simulink model "TDS_StateSpace"  (R2019b)
settings: Solver=VariableStepAuto  StartTime=0.0  StopTime=1500  RelTol=1e-3
values from neighbouring files (symbols this model uses):
  A = [0 -th2 th4; 0 -1/th3 0; 0 0 -1/th5]    [AP_TimeDelay.m]    (also in SmithControl.m; TimeDelayParameters.m = [0 -th2 0 th4 0; 0 -1/th3 1/th3 0 0; 0 0 -1/th3 0 0; 0 0 0 -; positivity_matrix.m; rscale.m = [0 -th2 0 th4 0; 0 -1/th3 1/th3 0 0; 0 0 -1/th3 0 0; 0 0 0 -)
  B = [0 0; 1/th3 0; 0 1/th5]    [AP_TimeDelay.m]    (also in SmithControl.m; TimeDelayParameters.m = [0 0; 0 0; 1/th3 0; 0 0; 0 1/th5]; positivity_matrix.m; rscale.m = [0 0; 0 0; 1/th3 0; 0 0; 0 1/th5])
  Ba = [0 ; 0 ; 1/th3 ; 0 ; 0]    [TimeDelayParameters.m]    (also in positivity_matrix.m = [th1; 0; 0])
  C = [1 1 1]    [AP_TimeDelay.m]    (also in SmithControl.m = [1 0 0]; TimeDelayParameters.m = [1 0 0 0 0]; positivity_matrix.m = [1 0 0]; rscale.m = [1 0 0 0 0])
  SF1 = [k/th2 -k*th3 (k*th5*th4)/(th2)]    [positivity_matrix.m]
  th1 = 0.85    [AP_TimeDelay.m]    (also in SmithControl.m; TimeDelayParameters.m = 0.32; positivity_matrix.m; rscale.m)
  th2 = 50    [AP_TimeDelay.m]    (also in SmithControl.m; TimeDelayParameters.m; positivity_matrix.m; rscale.m)
  th3 = 60    [AP_TimeDelay.m]    (also in SmithControl.m; TimeDelayParameters.m = 70; positivity_matrix.m; rscale.m)
libraries: dspsrcs4 x1
settings Model: Creator=akshita_jain  LastModifiedBy=akshita_jain

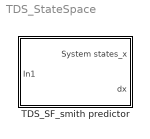
== system TDS_StateSpace ==
  TDS_SF_smith predictor : Subsystem

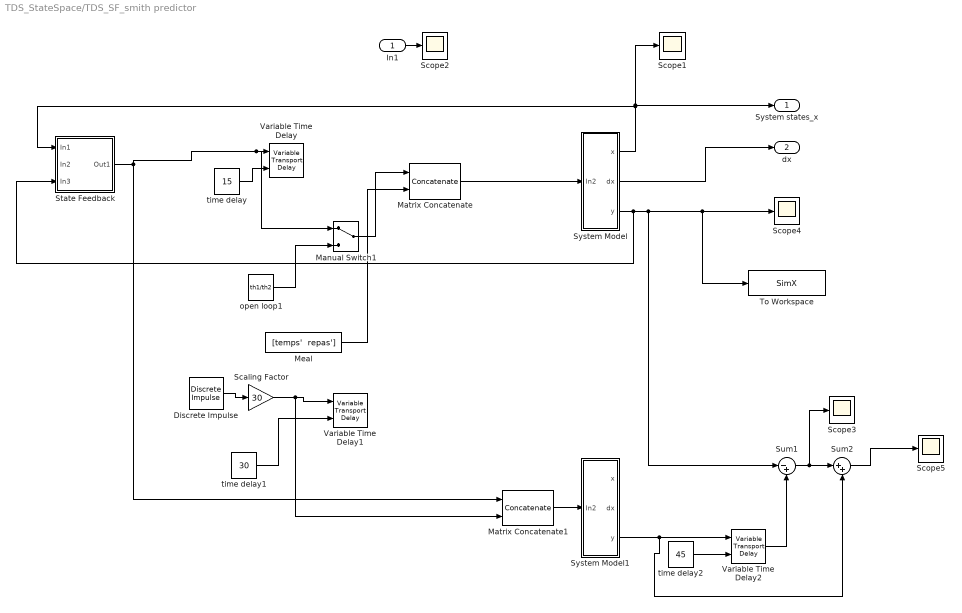
== system TDS_StateSpace/TDS_SF_smith predictor ==
  In1 : Inport
  Discrete Impulse : dspsrcs4/Discrete  Impulse  Delay=100  SampleTime=1  FrameSample=1  OutputFrames=off  dataType=double  isSigned=on  wordLen=16  udDataType=sfix(16)  fracBitsMode=Best precision  numFracBits=15  OutDataTypeStr=double  LastOutDataTypeStr=double
  Manual Switch1 : ManualSwitch
  Matrix Concatenate : Concatenate  ConcatenateDimension=2
  Matrix Concatenate1 : Concatenate  ConcatenateDimension=2
  Meal : FromWorkspace  VariableName="[temps'  repas']"  SampleTime=0
  Scaling Factor : Gain  Gain=30
  Scope{1..5} (5 alike) : Scope
  "State Feedback " : Subsystem
  Sum1 : Sum  Inputs=|-+
  Sum2 : Sum  Inputs=|++
  System Model : Subsystem
  System Model1 : Subsystem
  To Workspace : ToWorkspace  VariableName=SimX  SaveFormat=Timeseries  SampleTime=-1
  Variable Time Delay : VariableTransportDelay  MaximumDelay=20  InitialOutput=th1/th2
  Variable Time Delay1 : VariableTransportDelay  MaximumDelay=40  InitialOutput=0.00000000000001
  Variable Time Delay2 : VariableTransportDelay  MaximumDelay=60  InitialOutput=110
  open loop1 : Constant  Value=th1/th2
  time delay : Constant  Value=15  VectorParams1D=off
  time delay1 : Constant  Value=30  VectorParams1D=off
  time delay2 : Constant  Value=45  VectorParams1D=off
  System states_x : Outport
  dx : Outport  Port=2
  wires:
  time delay1/1 -> Variable Time Delay1/2
  Manual Switch1/1 -> Matrix Concatenate/1
  System Model/2(dx) -> dx/1
  time delay/1 -> Variable Time Delay/2
  open loop1/1 -> Manual Switch1/2
  Matrix Concatenate/1 -> System Model/1(In2)
  Scaling Factor/1 -> Matrix Concatenate1/2, Variable Time Delay1/1
  In1/1 -> Scope2/1
  System Model/1(x) -> System states_x/1, Scope1/1, "State Feedback "/1(In1)
  Discrete Impulse/1 -> Scaling Factor/1
  "State Feedback "/1(Out1) -> Manual Switch1/1, Variable Time Delay/1, Matrix Concatenate1/1
  System Model/3(y) -> "State Feedback "/3(In3), Sum1/1, To Workspace/1, Scope4/1
  System Model1/3(y) -> Sum2/2, Variable Time Delay2/1
  time delay2/1 -> Variable Time Delay2/2
  Variable Time Delay2/1 -> Sum1/2
  Sum1/1 -> Scope3/1, Sum2/1
  Sum2/1 -> Scope5/1
  Matrix Concatenate1/1 -> System Model1/1(In2)
  Meal/1 -> Matrix Concatenate/2

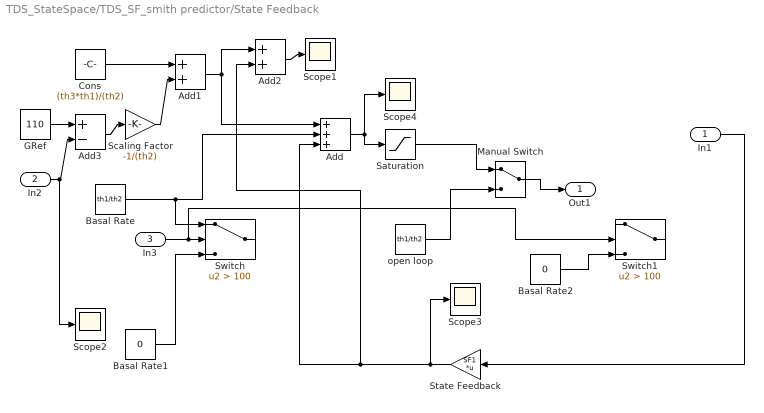
== system TDS_StateSpace/TDS_SF_smith predictor/State Feedback  ==
  In1 : Inport
  In2 : Inport  Port=2
  In3 : Inport  Port=3
  Add : Sum  Inputs=+++
  Add1 : Sum
  Add2 : Sum
  Add3 : Sum  Inputs=+-
  Basal Rate : Constant  Value=th1/th2  VectorParams1D=off
  Basal Rate1 : Constant  Value=0  VectorParams1D=off
  Basal Rate2 : Constant  Value=0  VectorParams1D=off
  Cons : Constant  Value=(th3*th1)/(th2)  VectorParams1D=off
  GRef : Constant  Value=110
  Manual Switch : ManualSwitch
  Saturation : Saturate  UpperLimit=2  LowerLimit=0
  Scaling Factor : Gain  Gain=-1/(th2)
  Scope{1..4} (4 alike) : Scope
  State Feedback : Gain  Gain=SF1  Multiplication=Matrix(K*u)
  Switch : Switch  Criteria=u2 > Threshold  Threshold=100
  Switch1 : Switch  Criteria=u2 > Threshold  Threshold=100
  open loop : Constant  Value=th1/th2
  Out1 : Outport
  wires:
  Manual Switch/1 -> Out1/1
  State Feedback/1 -> Add2/2, Add/3, Scope3/1
  In1/1 -> State Feedback/1
  Scaling Factor/1 -> Add1/2
  Add2/1 -> Scope1/1
  Add/1 -> Scope4/1, Saturation/1
  open loop/1 -> Manual Switch/2
  Saturation/1 -> Manual Switch/1
  Add1/1 -> Add/1, Add2/1
  Cons/1 -> Add1/1
  GRef/1 -> Add3/1
  Add3/1 -> Scaling Factor/1
  In2/1 -> Scope2/1, Add3/2
  Basal Rate/1 -> Add/2, Switch/1
  Basal Rate1/1 -> Switch/3
  In3/1 -> Switch1/2, Switch/2
  Basal Rate2/1 -> Switch1/3

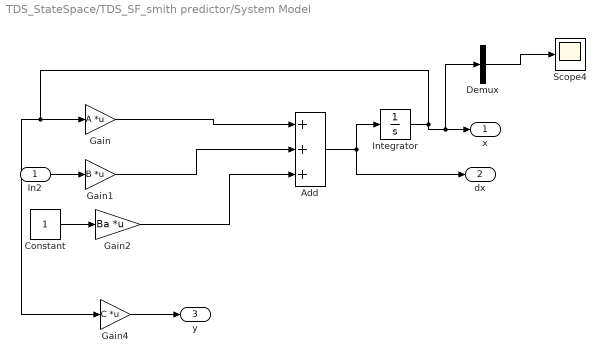
== system TDS_StateSpace/TDS_SF_smith predictor/System Model ==
  In2 : Inport
  Add : Sum  Inputs=3
  Constant : Constant
  Demux : Demux  Outputs=3
  Gain : Gain  Gain=A  Multiplication=Matrix(K*u)
  Gain1 : Gain  Gain=B  Multiplication=Matrix(K*u)
  Gain2 : Gain  Gain=Ba  Multiplication=Matrix(K*u)
  Gain4 : Gain  Gain=C  Multiplication=Matrix(K*u)
  Integrator : Integrator  InitialCondition=[110; th1/th2; 0]  ZeroCross=off
  Scope4 : Scope
  x : Outport
  dx : Outport  Port=2
  y : Outport  Port=3
  wires:
  Gain2/1 -> Add/3
  Gain1/1 -> Add/2
  Gain4/1 -> y/1
  Gain/1 -> Add/1
  Constant/1 -> Gain2/1
  In2/1 -> Gain1/1
  Add/1 -> dx/1, Integrator/1
  Integrator/1 -> Demux/1, x/1, Gain4/1, Gain/1
  Demux/2 -> Scope4/1

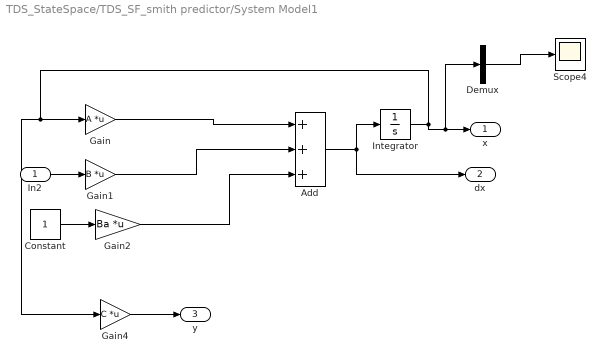
== system TDS_StateSpace/TDS_SF_smith predictor/System Model1 ==
  In2 : Inport
  Add : Sum  Inputs=3
  Constant : Constant
  Demux : Demux  Outputs=3
  Gain : Gain  Gain=A  Multiplication=Matrix(K*u)
  Gain1 : Gain  Gain=B  Multiplication=Matrix(K*u)
  Gain2 : Gain  Gain=Ba  Multiplication=Matrix(K*u)
  Gain4 : Gain  Gain=C  Multiplication=Matrix(K*u)
  Integrator : Integrator  InitialCondition=[110; th1/th2; 0]  ZeroCross=off
  Scope4 : Scope
  x : Outport
  dx : Outport  Port=2
  y : Outport  Port=3
  wires:
  Gain2/1 -> Add/3
  Gain1/1 -> Add/2
  Gain4/1 -> y/1
  Gain/1 -> Add/1
  Constant/1 -> Gain2/1
  In2/1 -> Gain1/1
  Add/1 -> dx/1, Integrator/1
  Integrator/1 -> Demux/1, x/1, Gain4/1, Gain/1
  Demux/2 -> Scope4/1
